simulink model "main"  (Simulink 8.0)
settings: Solver=ode4  StartTime=0.0  StopTime=stop_time  FixedStep=step_time  RelTol=1e-3
values from neighbouring files (symbols this model uses):
  alpha = 0.2    [main_1.m]
  Exp_Lamda = 7.9    [main_1.m]
  mean_wind = 10    [main_1.m]
  R = 38.5    [main_1.m]
libraries: wt_blockset_v3 x1
settings Model: Creator=dujiexian  LastModifiedBy=dujiexian

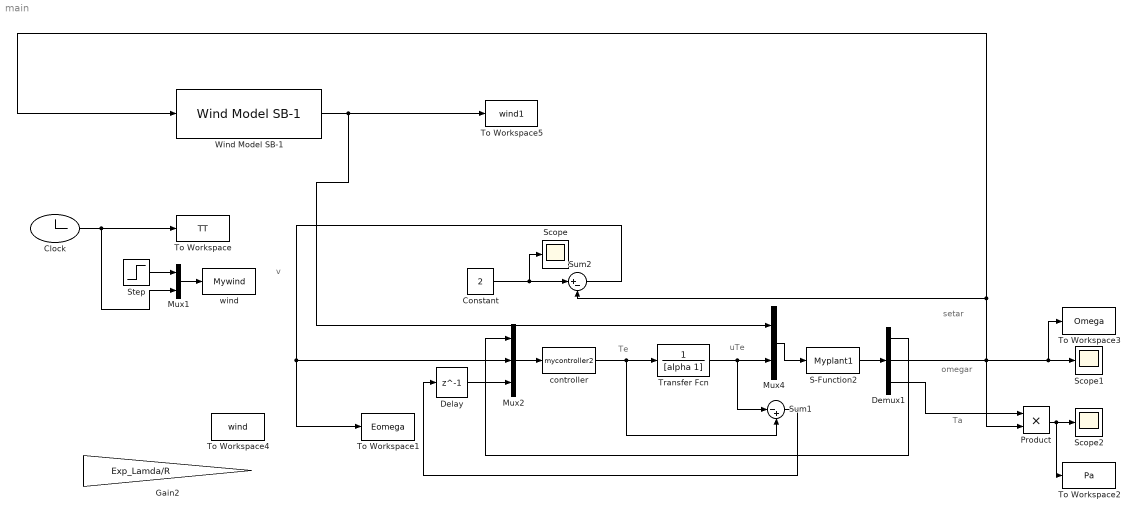
== system main ==
  note: Ta
  note: v
  note: Te
  note: uTe
  note: setar
  note: omegar
  Clock : Clock
  Constant : Constant  Value=2
  Delay : Delay  DelayLength=1  InitialCondition=0
  Demux1 : Demux  Outputs=3
  Gain2 : Gain  Gain=Exp_Lamda/R
  Mux1 : Mux  Inputs=2
  Mux2 : Mux  Inputs=3
  Mux4 : Mux  Inputs=2
  Product : Product  RndMeth=Zero
  S-Function2 : S-Function  FunctionName=Myplant1  EnableBusSupport=off
  Scope : Scope
      settings: YMin=2.25  YMax=2.675
  Scope1 : Scope
      settings: YMin=0  YMax=1.3
  Scope2 : Scope
      settings: YMin=0  YMax=1.3  SaveName=ScopeData2
  Step : Step  Time=0  After=mean_wind  SampleTime=0
  Sum1 : Sum  Inputs=|-+
  Sum2 : Sum  Inputs=|+-
  To Workspace : ToWorkspace  VariableName=TT  SampleTime=-1
  To Workspace1 : ToWorkspace  VariableName=Eomega  SampleTime=-1  SaveFormat=Timeseries
  To Workspace2 : ToWorkspace  VariableName=Pa  SampleTime=-1
  To Workspace3 : ToWorkspace  VariableName=Omega  SampleTime=-1
  To Workspace4 : ToWorkspace  VariableName=wind  SampleTime=-1
  To Workspace5 : ToWorkspace  VariableName=wind1  SampleTime=-1
  Transfer Fcn : TransferFcn  Denominator=[alpha 1]
  Wind Model SB-1 : wt_blockset_v3/Mechanical Components/Wind Model SB-1  D_rotor=72  v_mean=10  roughness=300  turb_int=12  T_sample=0.01
      link override Unit Delay: SampleTime=-1
      link override Unit Delay1: SampleTime=-1
  "controller " : MATLABFcn  MATLABFcn=mycontroller2  OutputDimensions=1  OutputSignalType=real
  wind : MATLABFcn  MATLABFcn=Mywind
  wires:
  Clock/1 -> To Workspace/1, Mux1/2
  Step/1 -> Mux1/1
  Mux1/1 -> wind/1
  "controller "/1 -> Sum1/2, Transfer Fcn/1
  S-Function2/1 -> Demux1/1
  Constant/1 -> Sum2/1, Scope/1
  Mux4/1 -> S-Function2/1
  Mux2/1 -> "controller "/1
  Transfer Fcn/1 -> Sum1/1, Mux4/2
  Sum2/1 -> Mux2/2, To Workspace1/1
  Demux1/1 -> Mux2/1
  Demux1/3 -> Product/1
  Product/1 -> To Workspace2/1, Scope2/1
  Demux1/2 -> Wind Model SB-1/1, Sum2/2, Product/2, To Workspace3/1, Scope1/1
  Wind Model SB-1/1 -> Mux4/1, To Workspace5/1
  Delay/1 -> Mux2/3
  Sum1/1 -> Delay/1
